simulink model "PubIfDecisionTOS_MDL"  (R2020b)
settings: configuration reference "DspaceConfig" (kept outside this file)
PostLoadFcn:
  | if any(exist('dsrtsu_mdlpostloadfcn', 'file') ~= 0), dsrtsu_mdlpostloadfcn('Execute', bdroot); end
InitFcn:
  | , if any(exist('dsmpb_private', 'file') ~= 0), dsmpb_private('dsmpb_mdlclblib', 'Init', bdroot); end,
undefined symbols (not defined in the file or in its folder): C_TOS_ACCEgoRAxletoFbumplength_m, C_TOS_ACCTargetFront_Flag, C_TOS_AEBJAPedObjDxThre_Val, C_TOS_AEBJAPedObjDyThre_Val, C_TOS_AEBJATargetSize_Val, C_TOS_AEBJAVehObjDxThre_Val, C_TOS_AEBJAVehObjDyThre_Val, C_TOS_AEBJuncPedTargetSize_Val, C_TOS_AEBLatObjDxThre_Val, C_TOS_AEBLatPedDyThre_Val, C_TOS_AEBLatTargetSize_Val, C_TOS_AEBLongTargetInEgoFront_Flag, C_TOS_axAbsGround_Parameter, C_TOS_CameraConfirmedFlag, C_TOS_CNsubjWidth, C_TOS_CurrentLaneCoreMinWidth_Val, C_TOS_CutInProb_Val_Zero, C_TOS_CutOutProb_Val_Zero, C_TOS_D2R_Val, C_TOS_DefaultValueObjectToCenterLine_dy, C_TOS_EgoCarWidth_Val, C_TOS_EgoDxRefPoint_m, C_TOS_EgoRAxletoFbumplength_m, C_TOS_HalfWidthVehicle_Con, C_TOS_HWA_CurrentLaneFlag, C_TOS_HWA_LeftLaneFlag, C_TOS_HWA_MovingDir_Vaild, C_TOS_HWA_MovState_Vaild, C_TOS_HWA_RightLaneFlag, C_TOS_LaneLineCourseErrorFront, C_TOS_LaneLineCourseErrorRear, C_TOS_MotorbikeDefaultWidth_m, C_TOS_NumberOfEffectiveTargets, C_TOS_Obj_Age_Val, C_TOS_Objdx_Constraint_Val, C_TOS_ObjectDefaultWidth_m, C_TOS_ObjInCurrentLane_Val, C_TOS_ObjInCurrentLaneValid, C_TOS_ObjInLeftLaneValid, C_TOS_ObjInRightLaneValid, C_TOS_ObjNotInCurrentLane_Val, C_TOS_ObjNotREElementType, C_TOS_ObjPredictDis_dy_ConstantVal_Zeros, C_TOS_ObjToCenterLine_ConstantVal_Zeros, C_TOS_OFMObjIDInvilad_Val, C_TOS_PIL_LatDisCons_Val_zero, C_TOS_PIL_ObjectCutInFlag_b, C_TOS_PIL_ObjectCutOutFlag_b, C_TOS_PIL_ObjLaneProb_al_Val, C_TOS_PP_ObjFusType_FC_Confirm_b, C_TOS_PP_ObjFusType_FC_FR_Confirm_b, C_TOS_PP_ObjFusType_FR_Confirm_b, C_TOS_RE_80BoolDefault_Val, C_TOS_RE_80Single181Default_Val, C_TOS_RE_80Single255Default_Val, C_TOS_RE_80Uint8Default_Val, C_TOS_RE_D2R, C_TOS_RE_D_180_Val, C_TOS_RE_InvalidObjectID_Val, C_TOS_RE_InvalidTargetChainDir_Val ... (+142)
libraries: simulink x1650, TOS_LIB x361, canfdmsglib x14
(part 23 of 69)

== system PubIfDecisionTOS_MDL/TOS_20201112/TOS_2012080320/PIL_1029/BoundaryCalculat/Lane_BoundaryCalculat/Lane_Boundary/Boundary/LeftLane_Boundary ==
  note: 用左侧车道虚拟出，左车道相邻车道
  Object_DX : Inport
  C_LaneLineCourseErrorFront : Inport  Port=2
  C_LaneLineCourseErrorRear : Inport  Port=3
  PP_CurrentLaneWidth : Inport  Port=4
  PP_LeftLaneWidth : Inport  Port=5
  SameLane_CoreArea_Boundary : Inport  Port=6
  LeftLane_BasicLaneWidth : Inport  Port=7
  Constant3 : Constant  Value=C_TOS_CurrentLaneCoreMinWidth_Val  OutDataTypeStr=single
      settings: AttributesFormatString=C_TOS_CurrentLaneCoreMinWidth_Val = 0
  Gain{,1..5} (6 alike) : Gain  Gain=0.5  ParamDataTypeStr=single  OutDataTypeStr=single
  Math Function : Math  Operator=square  SignedPower=on  OutDataTypeStr=single  SaturateOnIntegerOverflow=on
  MinMax : MinMax  Function=max  Inputs=2
  Product : Product  OutDataTypeStr=single
  Subtract : Sum  Inputs=+-  OutDataTypeStr=single
  Subtract1 : Sum  OutDataTypeStr=single
  Subtract2 : Sum  Inputs=+-  OutDataTypeStr=single
  Subtract3 : Sum  OutDataTypeStr=single
  Subtract4 : Sum  Inputs=+-  OutDataTypeStr=single
  Switch1 : Switch  OutDataTypeStr=single
  LeftLane_CoreArea_Boundary : Outport  OutDataTypeStr=single
  LeftLane_EdgeLeft_Boundary : Outport  Port=2
  LeftLane_EdgeRight_Boundary : Outport  Port=3
  wires:
  SameLane_CoreArea_Boundary/1 -> Subtract2/2
  Gain5/1 -> Subtract3/2
  Subtract4/1 -> LeftLane_EdgeLeft_Boundary/1
  Subtract3/1 -> Subtract4/1
  Gain4/1 -> Subtract3/1
  [LeftLane_CoreArea_Boundary] -> Subtract4/2
  PP_CurrentLaneWidth/1 -> Gain2/1
  Subtract1/1 -> Subtract2/1
  Gain3/1 -> Subtract1/2
  Gain2/1 -> Subtract1/1
  PP_LeftLaneWidth/1 -> Gain3/1, Gain4/1, Gain5/1
  Subtract2/1 -> LeftLane_EdgeRight_Boundary/1
  C_LaneLineCourseErrorRear/1 -> Switch1/3
  Switch1/1 -> Product/1
  Subtract/1 -> MinMax/1
  Gain1/1 -> Subtract/1
  LeftLane_BasicLaneWidth/1 -> Gain1/1
  Product/1 -> Subtract/2
  Math Function/1 -> Gain/1
  Gain/1 -> Product/2
  C_LaneLineCourseErrorFront/1 -> Switch1/1
  Object_DX/1 -> Math Function/1, Switch1/2
  Constant3/1 -> MinMax/2
  MinMax/1 -> LeftLane_CoreArea_Boundary/1, [LeftLane_CoreArea_Boundary]

== system PubIfDecisionTOS_MDL/TOS_20201112/TOS_2012080320/PIL_1029/BoundaryCalculat/Lane_BoundaryCalculat/Lane_Boundary/Boundary/RightLane_BasicLaneWidth ==
  ObjectType : Inport
  object_MovingState : Inport  Port=2
  PP_RightLaneWidth : Inport  Port=3
  Compare To Constant1 : simulink/Logic and Bit Operations/Compare To Constant  relop===  const=OFM_OBJ_TYPE_E.CAR  OutDataTypeStr=boolean
      settings: AttributesFormatString=OFM_OBJ_TYPE_E.CAR = 2
  Compare To Constant10 : simulink/Logic and Bit Operations/Compare To Constant  relop===  const=OFM_OBJ_MOVINGSTATE_E.UNKNOWN  OutDataTypeStr=boolean
      settings: AttributesFormatString=OFM_OBJ_MOVINGSTATE_E.UNKNOWN = 1
  Compare To Constant2 : simulink/Logic and Bit Operations/Compare To Constant  relop===  const=OFM_OBJ_TYPE_E.TRUCK  OutDataTypeStr=boolean
      settings: AttributesFormatString=OFM_OBJ_TYPE_E.TRUCK = 3
  Compare To Constant3 : simulink/Logic and Bit Operations/Compare To Constant  relop===  const=OFM_OBJ_TYPE_E.MOTORBIKE  OutDataTypeStr=boolean
      settings: AttributesFormatString=OFM_OBJ_TYPE_E.MOTORBIKE = 4
  Compare To Constant4 : simulink/Logic and Bit Operations/Compare To Constant  relop===  const=OFM_OBJ_TYPE_E.PEDESTRIAN  OutDataTypeStr=boolean
      settings: AttributesFormatString=OFM_OBJ_TYPE_E.PEDESTRIAN = 6
  Compare To Constant5 : simulink/Logic and Bit Operations/Compare To Constant  relop===  const=OFM_OBJ_TYPE_E.BICYCLE  OutDataTypeStr=boolean
      settings: AttributesFormatString=OFM_OBJ_TYPE_E.BICYCLE = 5
  Compare To Constant6 : simulink/Logic and Bit Operations/Compare To Constant  relop===  const=OFM_OBJ_TYPE_E.UNKNOWN_TYPE  OutDataTypeStr=boolean
      settings: AttributesFormatString=OFM_OBJ_TYPE_E.UNKNOWN_TYPE = 1
  Compare To Constant7 : simulink/Logic and Bit Operations/Compare To Constant  relop===  const=OFM_OBJ_TYPE_E.GENERAL_OBJECT  OutDataTypeStr=boolean
      settings: AttributesFormatString=OFM_OBJ_TYPE_E.GENERAL_OBJECT = 7
  Compare To Constant8 : simulink/Logic and Bit Operations/Compare To Constant  relop===  const=OFM_OBJ_TYPE_E.ANIMAL  OutDataTypeStr=boolean
      settings: AttributesFormatString=OFM_OBJ_TYPE_E.ANIMAL = 8
  Compare To Constant9 : simulink/Logic and Bit Operations/Compare To Constant  relop===  const=OFM_OBJ_MOVINGSTATE_E.STATIONARY  OutDataTypeStr=boolean
      settings: AttributesFormatString=OFM_OBJ_MOVINGSTATE_E.STATIONARY = 3
  Constant1 : Constant  Value=P_TOS_BasicLaneWidth_CAR_MinVal  OutDataTypeStr=single
      settings: AttributesFormatString=P_TOS_BasicLaneWidth_CAR_MinVal = 2.5
  Constant2 : Constant  Value=P_TOS_BasicLaneWidth_Pedestrian_MinVal  OutDataTypeStr=single
      settings: AttributesFormatString=P_TOS_BasicLaneWidth_Pedestrian_MinVal = 2
  Constant3 : Constant  Value=P_TOS_BasicLaneWidth_Bicycle_MinVal  OutDataTypeStr=single
      settings: AttributesFormatString=P_TOS_BasicLaneWidth_Bicycle_MinVal = 2.2
  Constant4 : Constant  Value=P_TOS_BasicLaneWidth_OthertType_MinVal  OutDataTypeStr=single
      settings: AttributesFormatString=P_TOS_BasicLaneWidth_OthertType_MinVal = 2.0
  Constant5 : Constant  Value=P_TOS_BasicLaneWidth_OthertType_MinVal  OutDataTypeStr=single
      settings: AttributesFormatString=P_TOS_BasicLaneWidth_OthertType_MinVal = 2.0
  Constant6 : Constant  Value=P_TOS_BasicLaneWidth_StillObj_MinVal  OutDataTypeStr=single
      settings: AttributesFormatString=P_TOS_BasicLaneWidth_StillObj_MinVal = 1.9
  Data Type Conversion : DataTypeConversion  OutDataTypeStr=Enum: OFM_OBJ_TYPE_E
  Data Type Conversion1 : DataTypeConversion  OutDataTypeStr=Enum: OFM_OBJ_MOVINGSTATE_E
  Logical Operator1 : Logic  Operator=OR  Inputs=3  AllPortsSameDT=off  OutDataTypeStr=boolean
  Logical Operator2 : Logic  Operator=OR  Inputs=3  AllPortsSameDT=off  OutDataTypeStr=boolean
  Logical Operator3 : Logic  Operator=OR  AllPortsSameDT=off  OutDataTypeStr=boolean
  MinMax : MinMax  Inputs=2  OutDataTypeStr=single
  Switch{1..5} (5 alike) : Switch  Criteria=u2 > Threshold
  RightLane_BasicLaneWidth : Outport
  wires:
  ObjectType/1 -> Data Type Conversion/1
  object_MovingState/1 -> Data Type Conversion1/1
  Compare To Constant4/1 -> Switch2/2
  Constant1/1 -> Switch1/1
  Constant3/1 -> Switch3/1
  Compare To Constant5/1 -> Switch3/2
  Constant5/1 -> Switch4/3
  Data Type Conversion/1 -> Compare To Constant1/1, Compare To Constant2/1, Compare To Constant6/1, Compare To Constant8/1, Compare To Constant7/1, Compare To Constant5/1, Compare To Constant4/1, Compare To Constant3/1
  Constant4/1 -> Switch4/1
  Constant2/1 -> Switch2/1
  Switch2/1 -> Switch1/3
  Switch4/1 -> Switch3/3
  Switch3/1 -> Switch2/3
  Compare To Constant3/1 -> Logical Operator1/3
  Switch1/1 -> Switch5/3
  Compare To Constant1/1 -> Logical Operator1/1
  Compare To Constant7/1 -> Logical Operator2/2
  Logical Operator2/1 -> Switch4/2
  Compare To Constant6/1 -> Logical Operator2/1
  Compare To Constant8/1 -> Logical Operator2/3
  Logical Operator1/1 -> Switch1/2
  Data Type Conversion1/1 -> Compare To Constant9/1, Compare To Constant10/1
  Compare To Constant2/1 -> Logical Operator1/2
  PP_RightLaneWidth/1 -> MinMax/1
  MinMax/1 -> RightLane_BasicLaneWidth/1
  Compare To Constant10/1 -> Logical Operator3/2
  Compare To Constant9/1 -> Logical Operator3/1
  Logical Operator3/1 -> Switch5/2
  Constant6/1 -> Switch5/1
  Switch5/1 -> MinMax/2

== system PubIfDecisionTOS_MDL/TOS_20201112/TOS_2012080320/PIL_1029/BoundaryCalculat/Lane_BoundaryCalculat/Lane_Boundary/Boundary/RightLane_Boundary ==
  note: 用右侧车道虚拟出，右车道相邻车道
  Object_DX : Inport
  C_LaneLineCourseErrorFront : Inport  Port=2
  C_LaneLineCourseErrorRear : Inport  Port=3
  PP_CurrentLaneWidth : Inport  Port=4
  PP_RightLaneWidth : Inport  Port=5
  SameLane_CoreArea_Boundary : Inport  Port=6
  RightLane_BasicLaneWidth : Inport  Port=7
  Constant3 : Constant  Value=C_TOS_CurrentLaneCoreMinWidth_Val  OutDataTypeStr=single
      settings: AttributesFormatString=C_TOS_CurrentLaneCoreMinWidth_Val = 0
  Gain{,1..5} (6 alike) : Gain  Gain=0.5  ParamDataTypeStr=single  OutDataTypeStr=single
  Math Function : Math  Operator=square  SignedPower=on  OutDataTypeStr=single  SaturateOnIntegerOverflow=on
  MinMax : MinMax  Function=max  Inputs=2
  Product : Product  OutDataTypeStr=single
  Subtract : Sum  Inputs=+-  OutDataTypeStr=single
  Subtract1 : Sum  OutDataTypeStr=single
  Subtract2 : Sum  Inputs=+-  OutDataTypeStr=single
  Subtract3 : Sum  OutDataTypeStr=single
  Subtract4 : Sum  Inputs=+-  OutDataTypeStr=single
  Switch1 : Switch  OutDataTypeStr=single
  RightLane_CoreArea_Boundary : Outport  OutDataTypeStr=single
  RightLane_EdgeLeft_Boundary : Outport  Port=2
  RightLane_EdgeRight_Boundary : Outport  Port=3
  wires:
  Subtract2/1 -> RightLane_EdgeLeft_Boundary/1
  Subtract4/1 -> RightLane_EdgeRight_Boundary/1
  Gain5/1 -> Subtract3/2
  PP_CurrentLaneWidth/1 -> Gain2/1
  Gain4/1 -> Subtract3/1
  PP_RightLaneWidth/1 -> Gain5/1, Gain4/1, Gain3/1
  Subtract3/1 -> Subtract4/1
  [RightLane_CoreArea_Boundary] -> Subtract4/2
  Subtract1/1 -> Subtract2/1
  Gain3/1 -> Subtract1/2
  Gain2/1 -> Subtract1/1
  SameLane_CoreArea_Boundary/1 -> Subtract2/2
  C_LaneLineCourseErrorRear/1 -> Switch1/3
  Switch1/1 -> Product/1
  Subtract/1 -> MinMax/1
  Gain1/1 -> Subtract/1
  RightLane_BasicLaneWidth/1 -> Gain1/1
  Product/1 -> Subtract/2
  Math Function/1 -> Gain/1
  Gain/1 -> Product/2
  C_LaneLineCourseErrorFront/1 -> Switch1/1
  Object_DX/1 -> Math Function/1, Switch1/2
  Constant3/1 -> MinMax/2
  MinMax/1 -> RightLane_CoreArea_Boundary/1, [RightLane_CoreArea_Boundary]

== system PubIfDecisionTOS_MDL/TOS_20201112/TOS_2012080320/PIL_1029/BoundaryCalculat/Lane_BoundaryCalculat/Lane_Boundary/Boundary/SameLane_BasicLaneWidth ==
  ObjectType : Inport
  object_MovingState : Inport  Port=2
  PP_CurrentLaneWidth : Inport  Port=3
  Compare To Constant1 : simulink/Logic and Bit Operations/Compare To Constant  relop===  const=OFM_OBJ_TYPE_E.CAR  OutDataTypeStr=boolean
      settings: AttributesFormatString=OFM_OBJ_TYPE_E.CAR = 2
  Compare To Constant10 : simulink/Logic and Bit Operations/Compare To Constant  relop===  const=OFM_OBJ_MOVINGSTATE_E.UNKNOWN  OutDataTypeStr=boolean
      settings: AttributesFormatString=OFM_OBJ_MOVINGSTATE_E.UNKNOWN = 1
  Compare To Constant2 : simulink/Logic and Bit Operations/Compare To Constant  relop===  const=OFM_OBJ_TYPE_E.TRUCK  OutDataTypeStr=boolean
      settings: AttributesFormatString=OFM_OBJ_TYPE_E.TRUCK = 3
  Compare To Constant3 : simulink/Logic and Bit Operations/Compare To Constant  relop===  const=OFM_OBJ_TYPE_E.MOTORBIKE  OutDataTypeStr=boolean
      settings: AttributesFormatString=OFM_OBJ_TYPE_E.MOTORBIKE = 4
  Compare To Constant4 : simulink/Logic and Bit Operations/Compare To Constant  relop===  const=OFM_OBJ_TYPE_E.PEDESTRIAN  OutDataTypeStr=boolean
      settings: AttributesFormatString=OFM_OBJ_TYPE_E.PEDESTRIAN = 6
  Compare To Constant5 : simulink/Logic and Bit Operations/Compare To Constant  relop===  const=OFM_OBJ_TYPE_E.BICYCLE  OutDataTypeStr=boolean
      settings: AttributesFormatString=OFM_OBJ_TYPE_E.BICYCLE = 5
  Compare To Constant6 : simulink/Logic and Bit Operations/Compare To Constant  relop===  const=OFM_OBJ_TYPE_E.UNKNOWN_TYPE  OutDataTypeStr=boolean
      settings: AttributesFormatString=OFM_OBJ_TYPE_E.UNKNOWN_TYPE = 1
  Compare To Constant7 : simulink/Logic and Bit Operations/Compare To Constant  relop===  const=OFM_OBJ_TYPE_E.GENERAL_OBJECT  OutDataTypeStr=boolean
      settings: AttributesFormatString=OFM_OBJ_TYPE_E.GENERAL_OBJECT = 7
  Compare To Constant8 : simulink/Logic and Bit Operations/Compare To Constant  relop===  const=OFM_OBJ_TYPE_E.ANIMAL  OutDataTypeStr=boolean
      settings: AttributesFormatString=OFM_OBJ_TYPE_E.ANIMAL = 8
  Compare To Constant9 : simulink/Logic and Bit Operations/Compare To Constant  relop===  const=OFM_OBJ_MOVINGSTATE_E.STATIONARY  OutDataTypeStr=boolean
      settings: AttributesFormatString=OFM_OBJ_MOVINGSTATE_E.STATIONARY = 3
  Constant1 : Constant  Value=P_TOS_BasicLaneWidth_CAR_MinVal  OutDataTypeStr=single
      settings: AttributesFormatString=P_TOS_BasicLaneWidth_CAR_MinVal = 2.5
  Constant2 : Constant  Value=P_TOS_BasicLaneWidth_Pedestrian_MinVal  OutDataTypeStr=single
      settings: AttributesFormatString=P_TOS_BasicLaneWidth_Pedestrian_MinVal = 2
  Constant3 : Constant  Value=P_TOS_BasicLaneWidth_Bicycle_MinVal  OutDataTypeStr=single
      settings: AttributesFormatString=P_TOS_BasicLaneWidth_Bicycle_MinVal = 2.2
  Constant4 : Constant  Value=P_TOS_BasicLaneWidth_OthertType_MinVal  OutDataTypeStr=single
      settings: AttributesFormatString=P_TOS_BasicLaneWidth_OthertType_MinVal = 2.0
  Constant5 : Constant  Value=P_TOS_BasicLaneWidth_OthertType_MinVal  OutDataTypeStr=single
      settings: AttributesFormatString=P_TOS_BasicLaneWidth_OthertType_MinVal = 2.0
  Constant6 : Constant  Value=P_TOS_BasicLaneWidth_StillObj_MinVal  OutDataTypeStr=single
      settings: AttributesFormatString=P_TOS_BasicLaneWidth_StillObj_MinVal = 1.9
  Data Type Conversion : DataTypeConversion  OutDataTypeStr=Enum: OFM_OBJ_TYPE_E
  Data Type Conversion1 : DataTypeConversion  OutDataTypeStr=Enum: OFM_OBJ_MOVINGSTATE_E
  Logical Operator1 : Logic  Operator=OR  Inputs=3  AllPortsSameDT=off  OutDataTypeStr=boolean
  Logical Operator2 : Logic  Operator=OR  Inputs=3  AllPortsSameDT=off  OutDataTypeStr=boolean
  Logical Operator3 : Logic  Operator=OR  AllPortsSameDT=off  OutDataTypeStr=boolean
  MinMax : MinMax  Inputs=2  OutDataTypeStr=single
  Switch{1..5} (5 alike) : Switch  Criteria=u2 > Threshold
  BasicLaneWidthOfCurrentLane : Outport
  wires:
  ObjectType/1 -> Data Type Conversion/1
  object_MovingState/1 -> Data Type Conversion1/1
  Compare To Constant4/1 -> Switch2/2
  Constant1/1 -> Switch1/1
  Constant3/1 -> Switch3/1
  Compare To Constant5/1 -> Switch3/2
  Constant5/1 -> Switch4/3
  Data Type Conversion/1 -> Compare To Constant1/1, Compare To Constant2/1, Compare To Constant6/1, Compare To Constant8/1, Compare To Constant7/1, Compare To Constant5/1, Compare To Constant4/1, Compare To Constant3/1
  Constant4/1 -> Switch4/1
  Constant2/1 -> Switch2/1
  Switch2/1 -> Switch1/3
  Switch4/1 -> Switch3/3
  Switch3/1 -> Switch2/3
  Compare To Constant3/1 -> Logical Operator1/3
  Switch1/1 -> Switch5/3
  Compare To Constant1/1 -> Logical Operator1/1
  Compare To Constant7/1 -> Logical Operator2/2
  Logical Operator2/1 -> Switch4/2
  Compare To Constant6/1 -> Logical Operator2/1
  Compare To Constant8/1 -> Logical Operator2/3
  Logical Operator1/1 -> Switch1/2
  Data Type Conversion1/1 -> Compare To Constant9/1, Compare To Constant10/1
  Compare To Constant2/1 -> Logical Operator1/2
  PP_CurrentLaneWidth/1 -> MinMax/1
  MinMax/1 -> BasicLaneWidthOfCurrentLane/1
  Compare To Constant10/1 -> Logical Operator3/2
  Compare To Constant9/1 -> Logical Operator3/1
  Logical Operator3/1 -> Switch5/2
  Constant6/1 -> Switch5/1
  Switch5/1 -> MinMax/2

== system PubIfDecisionTOS_MDL/TOS_20201112/TOS_2012080320/PIL_1029/BoundaryCalculat/Lane_BoundaryCalculat/Lane_Boundary/Boundary/SameLane_Boundary ==
  Object_DX : Inport
  C_LaneLineCourseErrorFront : Inport  Port=2
  C_LaneLineCourseErrorRear : Inport  Port=3
  PP_CurrentLaneWidth : Inport  Port=4
  PP_LeftLaneWidth : Inport  Port=5
  PP_RightLaneWidth : Inport  Port=6
  LeftLane_CoreArea_Boundary : Inport  Port=7
  RightLane_CoreArea_Boundary : Inport  Port=8
  SameLane_BasicLaneWidth : Inport  Port=9
  Constant3 : Constant  Value=C_TOS_CurrentLaneCoreMinWidth_Val  OutDataTypeStr=single
      settings: AttributesFormatString=C_TOS_CurrentLaneCoreMinWidth_Val = 0
  Gain{,1..5} (6 alike) : Gain  Gain=0.5  ParamDataTypeStr=single  OutDataTypeStr=single
  Math Function : Math  Operator=square  SignedPower=on  OutDataTypeStr=single  SaturateOnIntegerOverflow=on
  MinMax : MinMax  Function=max  Inputs=2
  Product : Product  OutDataTypeStr=single
  Subtract : Sum  Inputs=+-  OutDataTypeStr=single
  Subtract1 : Sum  OutDataTypeStr=single
  Subtract2 : Sum  Inputs=+-  OutDataTypeStr=single
  Subtract3 : Sum  OutDataTypeStr=single
  Subtract4 : Sum  Inputs=+-  OutDataTypeStr=single
  Switch1 : Switch  OutDataTypeStr=single
  SameLane_CoreArea_Boundary : Outport  OutDataTypeStr=single
  SameLane_EdgeLeft_Boundary : Outport  Port=2
  SameLane_EdgeRight_Boundary : Outport  Port=3
  wires:
  Subtract1/1 -> Subtract2/1
  PP_RightLaneWidth/1 -> Gain5/1
  Subtract2/1 -> SameLane_EdgeLeft_Boundary/1
  Gain3/1 -> Subtract1/2
  Gain5/1 -> Subtract3/2
  PP_CurrentLaneWidth/1 -> Gain4/1, Gain2/1
  LeftLane_CoreArea_Boundary/1 -> Subtract2/2
  Gain4/1 -> Subtract3/1
  Subtract4/1 -> SameLane_EdgeRight_Boundary/1
  Subtract3/1 -> Subtract4/1
  PP_LeftLaneWidth/1 -> Gain3/1
  RightLane_CoreArea_Boundary/1 -> Subtract4/2
  Gain2/1 -> Subtract1/1
  MinMax/1 -> SameLane_CoreArea_Boundary/1
  Constant3/1 -> MinMax/2
  Object_DX/1 -> Switch1/2, Math Function/1
  C_LaneLineCourseErrorFront/1 -> Switch1/1
  Gain/1 -> Product/2
  Math Function/1 -> Gain/1
  Product/1 -> Subtract/2
  SameLane_BasicLaneWidth/1 -> Gain1/1
  Gain1/1 -> Subtract/1
  Subtract/1 -> MinMax/1
  Switch1/1 -> Product/1
  C_LaneLineCourseErrorRear/1 -> Switch1/3

== system PubIfDecisionTOS_MDL/TOS_20201112/TOS_2012080320/PIL_1029/BoundaryCalculat/ObjectToCenterLine_dyc/LeftLane/LeftCenterLine_dyc/ObjToCenterLine_dyc_LeftLane ==
  Object_DY : Inport
  Object_DX : Inport  Port=2
  line01_C0 : Inport  Port=3
  line01_C1 : Inport  Port=4
  line01_C2 : Inport  Port=5
  line01_C3 : Inport  Port=6
  line01_dDisStart : Inport  Port=7
  line01_dDisEnd : Inport  Port=8
  line02_C0 : Inport  Port=9
  line02_C1 : Inport  Port=10
  line02_C2 : Inport  Port=11
  line02_C3 : Inport  Port=12
  line02_dDisStart : Inport  Port=13
  line02_dDisEnd : Inport  Port=14
  line03_C0 : Inport  Port=15
  line03_C1 : Inport  Port=16
  line03_C2 : Inport  Port=17
  line03_C3 : Inport  Port=18
  line03_dDisStart : Inport  Port=19
  line03_dDisEnd : Inport  Port=20
  line04_C0 : Inport  Port=21
  line04_C1 : Inport  Port=22
  line04_C2 : Inport  Port=23
  line04_C3 : Inport  Port=24
  line04_dDisStart : Inport  Port=25
  line04_dDisEnd : Inport  Port=26
  line05_C0 : Inport  Port=27
  line05_C1 : Inport  Port=28
  line05_C2 : Inport  Port=29
  line05_C3 : Inport  Port=30
  line05_dDisStart : Inport  Port=31
  line05_dDisEnd : Inport  Port=32
  line06_C0 : Inport  Port=33
  line06_C1 : Inport  Port=34
  line06_C2 : Inport  Port=35
  line06_C3 : Inport  Port=36
  line06_dDisStart : Inport  Port=37
  line06_dDisEnd : Inport  Port=38
  Action Port : ActionPort  ActionPortLabel=else
  Constant1 : Constant  Value=C_TOS_DefaultValueObjectToCenterLine_dy  OutDataTypeStr=single
      settings: AttributesFormatString=C_TOS_DefaultValueObjectToCenterLine_dy = 255
  Subtract : Sum  Inputs=+-
  Switch{,1..5} (6 alike) : Switch  Criteria=u2 ~= 0
  line01_DisJudge : Subsystem
  line01_dy : Subsystem
  line02_DisJudge : Subsystem
  line02_dy : Subsystem
  line03_DisJudge : Subsystem
  line03_dy : Subsystem
  line04_DisJudge : Subsystem
  line04_dy : Subsystem
  line05_DisJudge : Subsystem
  line05_dy : Subsystem
  line06_DisJudge : Subsystem
  line06_dy : Subsystem
  ObjectToCenterLine_dyc_LeftLane : Outport
  wires:
  Subtract/1 -> ObjectToCenterLine_dyc_LeftLane/1
  Object_DX/1 -> line01_dy/1(Object_DX), [Object_DX]
  line02_dDisEnd/1 -> line02_DisJudge/3(line02_dDisEnd)
  [Object_DX] -> line06_DisJudge/1(Object_DX)
  line05_dDisEnd/1 -> line05_DisJudge/3(line05_dDisEnd)
  line05_C0/1 -> line05_dy/2(line05_C0)
  line04_dDisEnd/1 -> line04_DisJudge/3(line04_dDisEnd)
  line06_dDisStart/1 -> line06_DisJudge/2(line06_dDisStart)
  line01_C0/1 -> line01_dy/2(line01_C0)
  [Object_DX] -> line05_DisJudge/1(Object_DX)
  [Object_DX] -> line04_DisJudge/1(Object_DX)
  line05_dy/1(line05_dy) -> Switch4/1
  [Object_DX] -> line01_DisJudge/1(Object_DX)
  line01_dDisEnd/1 -> line01_DisJudge/3(line01_dDisEnd)
  [Object_DX] -> line03_dy/1(Object_DX)
  line01_C1/1 -> line01_dy/3(line01_C1)
  line04_C0/1 -> line04_dy/2(line04_C0)
  line04_dDisStart/1 -> line04_DisJudge/2(line04_dDisStart)
  Constant1/1 -> Switch5/3
  line03_dDisStart/1 -> line03_DisJudge/2(line03_dDisStart)
  Switch/1 -> Subtract/2
  line02_dDisStart/1 -> line02_DisJudge/2(line02_dDisStart)
  line06_C3/1 -> line06_dy/5(line6_C3)
  line06_C0/1 -> line06_dy/2(line06_C0)
  line03_C1/1 -> line03_dy/3(line03_C1)
  line01_dDisStart/1 -> line01_DisJudge/2(line01_dDisStart)
  [Object_DX] -> line03_DisJudge/1(Object_DX)
  line06_C1/1 -> line06_dy/3(line06_C1)
  Switch5/1 -> Switch4/3
  line05_DisJudge/1(line05_DisJudge) -> Switch4/2
  line03_DisJudge/1(line03_DisJudge) -> Switch2/2
  line02_dy/1(line02_dy) -> Switch1/1
  line03_dy/1(line03_dy) -> Switch2/1
  line06_DisJudge/1(line06_DisJudge) -> Switch5/2
  Switch3/1 -> Switch2/3
  line04_dy/1(line04_dy) -> Switch3/1
  line02_C3/1 -> line02_dy/5(line02_C3)
  line04_DisJudge/1(line04_DisJudge) -> Switch3/2
  line04_C1/1 -> line04_dy/3(line04_C1)
  [Object_DX] -> line02_dy/1(Object_DX)
  line04_C3/1 -> line04_dy/5(line04_C3)
  line01_C2/1 -> line01_dy/4(line01_C2)
  line06_dDisEnd/1 -> line06_DisJudge/3(line06_dDisEnd)
  line01_DisJudge/1(line01_DisJudge) -> Switch/2
  Switch4/1 -> Switch3/3
  Object_DY/1 -> Subtract/1
  line01_dy/1(line01_dy) -> Switch/1
  [Object_DX] -> line02_DisJudge/1(Object_DX)
  line06_dy/1(line6_dy) -> Switch5/1
  line06_C2/1 -> line06_dy/4(line06_C2)
  line05_C1/1 -> line05_dy/3(line05_C1)
  line03_C2/1 -> line03_dy/4(line03_C2)
  line05_dDisStart/1 -> line05_DisJudge/2(line05_dDisStart)
  line02_C2/1 -> line02_dy/4(line02_C2)
  line02_C0/1 -> line02_dy/2(line02_C0)
  Switch2/1 -> Switch1/3
  line05_C3/1 -> line05_dy/5(line05_C3)
  [Object_DX] -> line06_dy/1(Object_DX)
  line03_dDisEnd/1 -> line03_DisJudge/3(line03_dDisEnd)
  line04_C2/1 -> line04_dy/4(line04_C2)
  Switch1/1 -> Switch/3
  [Object_DX] -> line04_dy/1(Object_DX)
  [Object_DX] -> line05_dy/1(Object_DX)
  line03_C3/1 -> line03_dy/5(line03_C3)
  line02_DisJudge/1(line02_DisJudge) -> Switch1/2
  line05_C2/1 -> line05_dy/4(line05_C2)
  line02_C1/1 -> line02_dy/3(line02_C1)
  line01_C3/1 -> line01_dy/5(line01_C3)
  line03_C0/1 -> line03_dy/2(line03_C0)

== system PubIfDecisionTOS_MDL/TOS_20201112/TOS_2012080320/PIL_1029/BoundaryCalculat/ObjectToCenterLine_dyc/LeftLane/LeftCenterLine_dyc/ObjToCenterLine_dyc_LeftLaneDefault ==
  Action Port : ActionPort  ActionPortLabel=if(u1 ~= 0)
  Constant2 : Constant  Value=255  OutDataTypeStr=single
  ObjectToCenterLine_dyc_LeftLane : Outport
  wires:
  Constant2/1 -> ObjectToCenterLine_dyc_LeftLane/1

== system PubIfDecisionTOS_MDL/TOS_20201112/TOS_2012080320/PIL_1029/BoundaryCalculat/ObjectToCenterLine_dyc/LeftLane/PIL_ObjectToCenterLine_dy_Filt/PIL_ObjectToCenterLine_dy ==
  ObjectID_Filt_K1 : Inport
  ObjectToCenterLine_dy_Filt_K1 : Inport  Port=2  OutDataTypeStr=single
  ObjectToCenterLine_dy : Inport  Port=3  OutDataTypeStr=single  Partition=on  PartitionDimension=1  PartitionWidth=1  PartitionOffset=0
  TOS_OFMObjValid_Flag : Inport  Port=4  OutDataTypeStr=uint8  Partition=on  PartitionDimension=1  PartitionWidth=1  PartitionOffset=0
  Object_ID : Inport  Port=5  OutDataTypeStr=uint8  Partition=on  PartitionDimension=1  PartitionWidth=1  PartitionOffset=0
  Object_Age : Inport  Port=6  Partition=on  PartitionDimension=1  PartitionWidth=1  PartitionOffset=0
  Compare To Constant : simulink/Logic and Bit Operations/Compare To Constant  relop===  const=C_TOS_OFMObjIDInvilad_Val  OutDataTypeStr=boolean
      settings: AttributesFormatString=C_TOS_OFMObjIDInvilad_Val = 0
  For Each : ForEach  DisableCoverage=on
  If : If  IfExpression=u1 ~= 0
  Merge : Merge
  Merge1 : Merge
  PP_SignalProcessingDefault : Subsystem  TreatAsAtomicUnit=on
  Subsystem : Subsystem
  Obj_ID : Outport  ConcatenationDimension=1
  ObjectToCenterLine_dy_Filt : Outport  Port=2  OutDataTypeStr=single  ConcatenationDimension=1
  wires:
  [TOS_OFMObjValid_Flag] -> Subsystem/6(TOS_OFMObjValid_Flag)
  TOS_OFMObjValid_Flag/1 -> Compare To Constant/1, [TOS_OFMObjValid_Flag]
  Object_Age/1 -> Subsystem/5(Object_Age)
  Merge/1 -> Obj_ID/1
  Merge1/1 -> ObjectToCenterLine_dy_Filt/1
  PP_SignalProcessingDefault/2(ObjectToCenterLine_dy_Filt) -> Merge1/1
  PP_SignalProcessingDefault/1(Obj_ID) -> Merge/1
  Subsystem/2(ObjectToCenterLine_dy_Filt) -> Merge1/2
  Subsystem/1(Obj_ID) -> Merge/2
  ObjectToCenterLine_dy/1 -> Subsystem/3(ObjectToCenterLine_dy)
  ObjectToCenterLine_dy_Filt_K1/1 -> Subsystem/2(ObjectToCenterLine_dy_Filt_K1)
  ObjectID_Filt_K1/1 -> Subsystem/1(ObjectID_Filt_K1)
  Compare To Constant/1 -> If/1
  Object_ID/1 -> Subsystem/4(Object_ID)
  If/1 -> PP_SignalProcessingDefault/Action
  If/2 -> Subsystem/Action

== system PubIfDecisionTOS_MDL/TOS_20201112/TOS_2012080320/PIL_1029/BoundaryCalculat/ObjectToCenterLine_dyc/RightLane/PIL_ObjectToCenterLine_dy_Filt/PIL_ObjectToCenterLine_dy ==
  ObjectID_Filt_K1 : Inport
  ObjectToCenterLine_dy_Filt_K1 : Inport  Port=2  OutDataTypeStr=single
  ObjectToCenterLine_dy : Inport  Port=3  OutDataTypeStr=single  Partition=on  PartitionDimension=1  PartitionWidth=1  PartitionOffset=0
  TOS_OFMObjValid_Flag : Inport  Port=4  OutDataTypeStr=uint8  Partition=on  PartitionDimension=1  PartitionWidth=1  PartitionOffset=0
  Object_ID : Inport  Port=5  OutDataTypeStr=uint8  Partition=on  PartitionDimension=1  PartitionWidth=1  PartitionOffset=0
  Object_Age : Inport  Port=6  Partition=on  PartitionDimension=1  PartitionWidth=1  PartitionOffset=0
  Compare To Constant : simulink/Logic and Bit Operations/Compare To Constant  relop===  const=C_TOS_OFMObjIDInvilad_Val  OutDataTypeStr=boolean
      settings: AttributesFormatString=C_TOS_OFMObjIDInvilad_Val = 0
  For Each : ForEach  DisableCoverage=on
  If : If  IfExpression=u1 ~= 0
  Merge : Merge
  Merge1 : Merge
  PP_SignalProcessingDefault : Subsystem  TreatAsAtomicUnit=on
  Subsystem : Subsystem
  Obj_ID : Outport  ConcatenationDimension=1
  ObjectToCenterLine_dy_Filt : Outport  Port=2  OutDataTypeStr=single  ConcatenationDimension=1
  wires:
  [TOS_OFMObjValid_Flag] -> Subsystem/6(TOS_OFMObjValid_Flag)
  TOS_OFMObjValid_Flag/1 -> Compare To Constant/1, [TOS_OFMObjValid_Flag]
  Object_Age/1 -> Subsystem/5(Object_Age)
  Merge/1 -> Obj_ID/1
  Merge1/1 -> ObjectToCenterLine_dy_Filt/1
  PP_SignalProcessingDefault/2(ObjectToCenterLine_dy_Filt) -> Merge1/1
  PP_SignalProcessingDefault/1(Obj_ID) -> Merge/1
  Subsystem/2(ObjectToCenterLine_dy_Filt) -> Merge1/2
  Subsystem/1(Obj_ID) -> Merge/2
  ObjectToCenterLine_dy/1 -> Subsystem/3(ObjectToCenterLine_dy)
  ObjectToCenterLine_dy_Filt_K1/1 -> Subsystem/2(ObjectToCenterLine_dy_Filt_K1)
  ObjectID_Filt_K1/1 -> Subsystem/1(ObjectID_Filt_K1)
  Compare To Constant/1 -> If/1
  Object_ID/1 -> Subsystem/4(Object_ID)
  If/1 -> PP_SignalProcessingDefault/Action
  If/2 -> Subsystem/Action

== system PubIfDecisionTOS_MDL/TOS_20201112/TOS_2012080320/PIL_1029/BoundaryCalculat/ObjectToCenterLine_dyc/RightLane/RightCenterLine_dyc/ObjToCenterLine_dyc_RightLane ==
  Object_DY : Inport
  Object_DX : Inport  Port=2
  line01_C0 : Inport  Port=3
  line01_C1 : Inport  Port=4
  line01_C2 : Inport  Port=5
  line01_C3 : Inport  Port=6
  line01_dDisStart : Inport  Port=7
  line01_dDisEnd : Inport  Port=8
  line02_C0 : Inport  Port=9
  line02_C1 : Inport  Port=10
  line02_C2 : Inport  Port=11
  line02_C3 : Inport  Port=12
  line02_dDisStart : Inport  Port=13
  line02_dDisEnd : Inport  Port=14
  line03_C0 : Inport  Port=15
  line03_C1 : Inport  Port=16
  line03_C2 : Inport  Port=17
  line03_C3 : Inport  Port=18
  line03_dDisStart : Inport  Port=19
  line03_dDisEnd : Inport  Port=20
  line04_C0 : Inport  Port=21
  line04_C1 : Inport  Port=22
  line04_C2 : Inport  Port=23
  line04_C3 : Inport  Port=24
  line04_dDisStart : Inport  Port=25
  line04_dDisEnd : Inport  Port=26
  line05_C0 : Inport  Port=27
  line05_C1 : Inport  Port=28
  line05_C2 : Inport  Port=29
  line05_C3 : Inport  Port=30
  line05_dDisStart : Inport  Port=31
  line05_dDisEnd : Inport  Port=32
  line06_C0 : Inport  Port=33
  line06_C1 : Inport  Port=34
  line06_C2 : Inport  Port=35
  line06_C3 : Inport  Port=36
  line06_dDisStart : Inport  Port=37
  line06_dDisEnd : Inport  Port=38
  Action Port : ActionPort  ActionPortLabel=else
  Constant1 : Constant  Value=C_TOS_DefaultValueObjectToCenterLine_dy  OutDataTypeStr=single
      settings: AttributesFormatString=C_TOS_DefaultValueObjectToCenterLine_dy = 255
  Subtract : Sum  Inputs=+-
  Switch{,1..5} (6 alike) : Switch  Criteria=u2 ~= 0
  line01_DisJudge : Subsystem
  line01_dy : Subsystem
  line02_DisJudge : Subsystem
  line02_dy : Subsystem
  line03_DisJudge : Subsystem
  line03_dy : Subsystem
  line04_DisJudge : Subsystem
  line04_dy : Subsystem
  line05_DisJudge : Subsystem
  line05_dy : Subsystem
  line06_DisJudge : Subsystem
  line06_dy : Subsystem
  ObjectToCenterLine_dyc_RightLane : Outport
  wires:
  line03_C0/1 -> line03_dy/2(line03_C0)
  line01_C3/1 -> line01_dy/5(line01_C3)
  line02_C1/1 -> line02_dy/3(line02_C1)
  line05_C2/1 -> line05_dy/4(line05_C2)
  line02_DisJudge/1(line02_DisJudge) -> Switch1/2
  line03_C3/1 -> line03_dy/5(line03_C3)
  [Object_DX] -> line05_dy/1(Object_DX)
  [Object_DX] -> line04_dy/1(Object_DX)
  Switch1/1 -> Switch/3
  line04_C2/1 -> line04_dy/4(line04_C2)
  line03_dDisEnd/1 -> line03_DisJudge/3(line03_dDisEnd)
  [Object_DX] -> line06_dy/1(Object_DX)
  line05_C3/1 -> line05_dy/5(line05_C3)
  Switch2/1 -> Switch1/3
  line02_C0/1 -> line02_dy/2(line02_C0)
  line02_C2/1 -> line02_dy/4(line02_C2)
  line05_dDisStart/1 -> line05_DisJudge/2(line05_dDisStart)
  line03_C2/1 -> line03_dy/4(line03_C2)
  line05_C1/1 -> line05_dy/3(line05_C1)
  line06_C2/1 -> line06_dy/4(line06_C2)
  line06_dy/1(line6_dy) -> Switch5/1
  [Object_DX] -> line02_DisJudge/1(Object_DX)
  line01_dy/1(line01_dy) -> Switch/1
  Object_DY/1 -> Subtract/1
  Switch4/1 -> Switch3/3
  line01_DisJudge/1(line01_DisJudge) -> Switch/2
  line06_dDisEnd/1 -> line06_DisJudge/3(line06_dDisEnd)
  line01_C2/1 -> line01_dy/4(line01_C2)
  line04_C3/1 -> line04_dy/5(line04_C3)
  [Object_DX] -> line02_dy/1(Object_DX)
  line04_C1/1 -> line04_dy/3(line04_C1)
  line04_DisJudge/1(line04_DisJudge) -> Switch3/2
  line02_C3/1 -> line02_dy/5(line02_C3)
  line04_dy/1(line04_dy) -> Switch3/1
  Switch3/1 -> Switch2/3
  line06_DisJudge/1(line06_DisJudge) -> Switch5/2
  line03_dy/1(line03_dy) -> Switch2/1
  line02_dy/1(line02_dy) -> Switch1/1
  line03_DisJudge/1(line03_DisJudge) -> Switch2/2
  line05_DisJudge/1(line05_DisJudge) -> Switch4/2
  Switch5/1 -> Switch4/3
  line06_C1/1 -> line06_dy/3(line06_C1)
  [Object_DX] -> line03_DisJudge/1(Object_DX)
  line01_dDisStart/1 -> line01_DisJudge/2(line01_dDisStart)
  line03_C1/1 -> line03_dy/3(line03_C1)
  line06_C0/1 -> line06_dy/2(line06_C0)
  line06_C3/1 -> line06_dy/5(line6_C3)
  line02_dDisStart/1 -> line02_DisJudge/2(line02_dDisStart)
  Switch/1 -> Subtract/2
  line03_dDisStart/1 -> line03_DisJudge/2(line03_dDisStart)
  Constant1/1 -> Switch5/3
  line04_dDisStart/1 -> line04_DisJudge/2(line04_dDisStart)
  line04_C0/1 -> line04_dy/2(line04_C0)
  line01_C1/1 -> line01_dy/3(line01_C1)
  [Object_DX] -> line03_dy/1(Object_DX)
  line01_dDisEnd/1 -> line01_DisJudge/3(line01_dDisEnd)
  [Object_DX] -> line01_DisJudge/1(Object_DX)
  line05_dy/1(line05_dy) -> Switch4/1
  [Object_DX] -> line04_DisJudge/1(Object_DX)
  [Object_DX] -> line05_DisJudge/1(Object_DX)
  line01_C0/1 -> line01_dy/2(line01_C0)
  line06_dDisStart/1 -> line06_DisJudge/2(line06_dDisStart)
  line04_dDisEnd/1 -> line04_DisJudge/3(line04_dDisEnd)
  line05_C0/1 -> line05_dy/2(line05_C0)
  line05_dDisEnd/1 -> line05_DisJudge/3(line05_dDisEnd)
  [Object_DX] -> line06_DisJudge/1(Object_DX)
  line02_dDisEnd/1 -> line02_DisJudge/3(line02_dDisEnd)
  Object_DX/1 -> [Object_DX], line01_dy/1(Object_DX)
  Subtract/1 -> ObjectToCenterLine_dyc_RightLane/1

== system PubIfDecisionTOS_MDL/TOS_20201112/TOS_2012080320/PIL_1029/BoundaryCalculat/ObjectToCenterLine_dyc/RightLane/RightCenterLine_dyc/ObjToCenterLine_dyc_RightLaneDefault ==
  Action Port : ActionPort  ActionPortLabel=if(u1 ~= 0)
  Constant2 : Constant  Value=255  OutDataTypeStr=single
  ObjectToCenterLine_dyc_LeftLane : Outport
  wires:
  Constant2/1 -> ObjectToCenterLine_dyc_LeftLane/1

== system PubIfDecisionTOS_MDL/TOS_20201112/TOS_2012080320/PIL_1029/BoundaryCalculat/ObjectToCenterLine_dyc/SameLane/PIL_ObjectToCenterLine_dy_Filt/PIL_ObjectToCenterLine_dy ==
  ObjectID_Filt_K1 : Inport
  ObjectToCenterLine_dy_Filt_K1 : Inport  Port=2  OutDataTypeStr=single
  ObjectToCenterLine_dy : Inport  Port=3  OutDataTypeStr=single  Partition=on  PartitionDimension=1  PartitionWidth=1  PartitionOffset=0
  TOS_OFMObjValid_Flag : Inport  Port=4  OutDataTypeStr=uint8  Partition=on  PartitionDimension=1  PartitionWidth=1  PartitionOffset=0
  Object_ID : Inport  Port=5  OutDataTypeStr=uint8  Partition=on  PartitionDimension=1  PartitionWidth=1  PartitionOffset=0
  Object_Age : Inport  Port=6  Partition=on  PartitionDimension=1  PartitionWidth=1  PartitionOffset=0
  Compare To Constant : simulink/Logic and Bit Operations/Compare To Constant  relop===  const=C_TOS_OFMObjIDInvilad_Val  OutDataTypeStr=boolean
      settings: AttributesFormatString=C_TOS_OFMObjIDInvilad_Val = 0
  For Each : ForEach  DisableCoverage=on
  If : If  IfExpression=u1 ~= 0
  Merge : Merge
  Merge1 : Merge
  PP_SignalProcessingDefault : Subsystem  TreatAsAtomicUnit=on
  Subsystem : Subsystem
  Obj_ID : Outport  ConcatenationDimension=1
  ObjectToCenterLine_dy_Filt : Outport  Port=2  OutDataTypeStr=single  ConcatenationDimension=1
  wires:
  [TOS_OFMObjValid_Flag] -> Subsystem/6(TOS_OFMObjValid_Flag)
  TOS_OFMObjValid_Flag/1 -> Compare To Constant/1, [TOS_OFMObjValid_Flag]
  Object_Age/1 -> Subsystem/5(Object_Age)
  Merge/1 -> Obj_ID/1
  Merge1/1 -> ObjectToCenterLine_dy_Filt/1
  PP_SignalProcessingDefault/2(ObjectToCenterLine_dy_Filt) -> Merge1/1
  PP_SignalProcessingDefault/1(Obj_ID) -> Merge/1
  Subsystem/2(ObjectToCenterLine_dy_Filt) -> Merge1/2
  Subsystem/1(Obj_ID) -> Merge/2
  ObjectToCenterLine_dy/1 -> Subsystem/3(ObjectToCenterLine_dy)
  ObjectToCenterLine_dy_Filt_K1/1 -> Subsystem/2(ObjectToCenterLine_dy_Filt_K1)
  ObjectID_Filt_K1/1 -> Subsystem/1(ObjectID_Filt_K1)
  Compare To Constant/1 -> If/1
  Object_ID/1 -> Subsystem/4(Object_ID)
  If/1 -> PP_SignalProcessingDefault/Action
  If/2 -> Subsystem/Action

== system PubIfDecisionTOS_MDL/TOS_20201112/TOS_2012080320/PIL_1029/BoundaryCalculat/ObjectToCenterLine_dyc/SameLane/SameCenterLine_dyc/ObjToCenterLine_dyc_CurrentLane ==
  Object_DY : Inport
  Object_DX : Inport  Port=2
  line01_C0 : Inport  Port=3
  line01_C1 : Inport  Port=4
  line01_C2 : Inport  Port=5
  line01_C3 : Inport  Port=6
  line01_dDisStart : Inport  Port=7
  line01_dDisEnd : Inport  Port=8
  line02_C0 : Inport  Port=9
  line02_C1 : Inport  Port=10
  line02_C2 : Inport  Port=11
  line02_C3 : Inport  Port=12
  line02_dDisStart : Inport  Port=13
  line02_dDisEnd : Inport  Port=14
  line03_C0 : Inport  Port=15
  line03_C1 : Inport  Port=16
  line03_C2 : Inport  Port=17
  line03_C3 : Inport  Port=18
  line03_dDisStart : Inport  Port=19
  line03_dDisEnd : Inport  Port=20
  line04_C0 : Inport  Port=21
  line04_C1 : Inport  Port=22
  line04_C2 : Inport  Port=23
  line04_C3 : Inport  Port=24
  line04_dDisStart : Inport  Port=25
  line04_dDisEnd : Inport  Port=26
  line05_C0 : Inport  Port=27
  line05_C1 : Inport  Port=28
  line05_C2 : Inport  Port=29
  line05_C3 : Inport  Port=30
  line05_dDisStart : Inport  Port=31
  line05_dDisEnd : Inport  Port=32
  line06_C0 : Inport  Port=33
  line06_C1 : Inport  Port=34
  line06_C2 : Inport  Port=35
  line06_C3 : Inport  Port=36
  line06_dDisStart : Inport  Port=37
  line06_dDisEnd : Inport  Port=38
  Action Port : ActionPort  ActionPortLabel=else
  Constant1 : Constant  Value=C_TOS_DefaultValueObjectToCenterLine_dy  OutDataTypeStr=single
      settings: AttributesFormatString=C_TOS_DefaultValueObjectToCenterLine_dy = 255
  Subtract : Sum  Inputs=+-
  Switch{,1..5} (6 alike) : Switch  Criteria=u2 ~= 0
  line01_DisJudge : Subsystem
  line01_dy : Subsystem
  line02_DisJudge : Subsystem
  line02_dy : Subsystem
  line03_DisJudge : Subsystem
  line03_dy : Subsystem
  line04_DisJudge : Subsystem
  line04_dy : Subsystem
  line05_DisJudge : Subsystem
  line05_dy : Subsystem
  line06_DisJudge : Subsystem
  line06_dy : Subsystem
  ObjectToCenterLine_dyc_CurrentLane : Outport
  wires:
  Subtract/1 -> ObjectToCenterLine_dyc_CurrentLane/1
  Object_DX/1 -> line01_dy/1(Object_DX), [Object_DX]
  line02_dDisEnd/1 -> line02_DisJudge/3(line02_dDisEnd)
  [Object_DX] -> line06_DisJudge/1(Object_DX)
  line05_dDisEnd/1 -> line05_DisJudge/3(line05_dDisEnd)
  line05_C0/1 -> line05_dy/2(line05_C0)
  line04_dDisEnd/1 -> line04_DisJudge/3(line04_dDisEnd)
  line06_dDisStart/1 -> line06_DisJudge/2(line06_dDisStart)
  line01_C0/1 -> line01_dy/2(line01_C0)
  [Object_DX] -> line05_DisJudge/1(Object_DX)
  [Object_DX] -> line04_DisJudge/1(Object_DX)
  line05_dy/1(line05_dy) -> Switch4/1
  [Object_DX] -> line01_DisJudge/1(Object_DX)
  line01_dDisEnd/1 -> line01_DisJudge/3(line01_dDisEnd)
  [Object_DX] -> line03_dy/1(Object_DX)
  line01_C1/1 -> line01_dy/3(line01_C1)
  line04_C0/1 -> line04_dy/2(line04_C0)
  line04_dDisStart/1 -> line04_DisJudge/2(line04_dDisStart)
  Constant1/1 -> Switch5/3
  line03_dDisStart/1 -> line03_DisJudge/2(line03_dDisStart)
  Switch/1 -> Subtract/2
  line02_dDisStart/1 -> line02_DisJudge/2(line02_dDisStart)
  line06_C3/1 -> line06_dy/5(line6_C3)
  line06_C0/1 -> line06_dy/2(line06_C0)
  line03_C1/1 -> line03_dy/3(line03_C1)
  line01_dDisStart/1 -> line01_DisJudge/2(line01_dDisStart)
  [Object_DX] -> line03_DisJudge/1(Object_DX)
  line06_C1/1 -> line06_dy/3(line06_C1)
  Switch5/1 -> Switch4/3
  line05_DisJudge/1(line05_DisJudge) -> Switch4/2
  line03_DisJudge/1(line03_DisJudge) -> Switch2/2
  line02_dy/1(line02_dy) -> Switch1/1
  line03_dy/1(line03_dy) -> Switch2/1
  line06_DisJudge/1(line06_DisJudge) -> Switch5/2
  Switch3/1 -> Switch2/3
  line04_dy/1(line04_dy) -> Switch3/1
  line02_C3/1 -> line02_dy/5(line02_C3)
  line04_DisJudge/1(line04_DisJudge) -> Switch3/2
  line04_C1/1 -> line04_dy/3(line04_C1)
  [Object_DX] -> line02_dy/1(Object_DX)
  line04_C3/1 -> line04_dy/5(line04_C3)
  line01_C2/1 -> line01_dy/4(line01_C2)
  line06_dDisEnd/1 -> line06_DisJudge/3(line06_dDisEnd)
  line01_DisJudge/1(line01_DisJudge) -> Switch/2
  Switch4/1 -> Switch3/3
  Object_DY/1 -> Subtract/1
  line01_dy/1(line01_dy) -> Switch/1
  [Object_DX] -> line02_DisJudge/1(Object_DX)
  line06_dy/1(line6_dy) -> Switch5/1
  line06_C2/1 -> line06_dy/4(line06_C2)
  line05_C1/1 -> line05_dy/3(line05_C1)
  line03_C2/1 -> line03_dy/4(line03_C2)
  line05_dDisStart/1 -> line05_DisJudge/2(line05_dDisStart)
  line02_C2/1 -> line02_dy/4(line02_C2)
  line02_C0/1 -> line02_dy/2(line02_C0)
  Switch2/1 -> Switch1/3
  line05_C3/1 -> line05_dy/5(line05_C3)
  [Object_DX] -> line06_dy/1(Object_DX)
  line03_dDisEnd/1 -> line03_DisJudge/3(line03_dDisEnd)
  line04_C2/1 -> line04_dy/4(line04_C2)
  Switch1/1 -> Switch/3
  [Object_DX] -> line04_dy/1(Object_DX)
  [Object_DX] -> line05_dy/1(Object_DX)
  line03_C3/1 -> line03_dy/5(line03_C3)
  line02_DisJudge/1(line02_DisJudge) -> Switch1/2
  line05_C2/1 -> line05_dy/4(line05_C2)
  line02_C1/1 -> line02_dy/3(line02_C1)
  line01_C3/1 -> line01_dy/5(line01_C3)
  line03_C0/1 -> line03_dy/2(line03_C0)

== system PubIfDecisionTOS_MDL/TOS_20201112/TOS_2012080320/PIL_1029/BoundaryCalculat/ObjectToCenterLine_dyc/SameLane/SameCenterLine_dyc/ObjToCenterLine_dyc_CurrentLaneDefault ==
  Action Port : ActionPort  ActionPortLabel=if(u1 ~= 0)
  Constant2 : Constant  Value=255  OutDataTypeStr=single
  ObjectToCenterLine_dyc_CurrentLane : Outport
  wires:
  Constant2/1 -> ObjectToCenterLine_dyc_CurrentLane/1

== system PubIfDecisionTOS_MDL/TOS_20201112/TOS_2012080320/PIL_1029/ObjCutInOut_Prob/ObjectCutIn/CutInProb_Calculate/CutInProb_Calculate_/CutInPredictDis_dy ==
  note: dx 修正vyc的 cut in 预测时间
  ObjectToCenterLine_dy_Filt : Inport  OutDataTypeStr=single
  ObjectToCenterLine_dy : Inport  Port=2  OutDataTypeStr=single
  ObjectType : Inport  Port=3
  Object_DX : Inport  Port=4
  PP_ObjectToCenterLine_vyc : Inport  Port=5
  CutInPredictTime : Subsystem
  CutInPredictTime_Constraint : Subsystem
  CutInPredictTime_Constraint2 : Subsystem
  PIL_CutInPredictTime_ObserVale : Outport  OutDataTypeStr=single
  PIL_CutInPredictTime_Constraint_ObserVale : Outport  Port=2  OutDataTypeStr=single
  CutInPredictDis_dy : Outport  Port=3  OutDataTypeStr=single
  wires:
  Object_DX/1 -> CutInPredictTime/5(Object_DX), CutInPredictTime_Constraint/2(Object_DX)
  ObjectToCenterLine_dy_Filt/1 -> CutInPredictTime/1(ObjectToCenterLine_dy_Filt)
  ObjectToCenterLine_dy/1 -> [ObjectToCenterLine_dy], CutInPredictTime/2(ObjectToCenterLine_dy)
  CutInPredictTime/1(CutInPredictTime) -> [PIL_CutInPredictTime_ObserVale], CutInPredictTime_Constraint/1(CutInPredictTime)
  CutInPredictTime_Constraint/1(CutInPredictTime_Constraint) -> [PIL_CutInPredictTime_Constraint_ObserVale], CutInPredictTime_Constraint2/2(CutInPredictTime_Constraint)
  PP_ObjectToCenterLine_vyc/1 -> CutInPredictTime_Constraint2/3(PP_ObjectToCenterLine_vyc), [PP_ObjectToCenterLine_vyc]
  CutInPredictTime_Constraint2/1(CutInPredictDis_dy) -> CutInPredictDis_dy/1
  [ObjectToCenterLine_dy] -> CutInPredictTime_Constraint2/1(ObjectToCenterLine_dy)
  ObjectType/1 -> CutInPredictTime/3(ObjectType)
  [PP_ObjectToCenterLine_vyc] -> CutInPredictTime/4(PP_ObjectToCenterLine_vyc)
  [PIL_CutInPredictTime_Constraint_ObserVale] -> PIL_CutInPredictTime_Constraint_ObserVale/1
  [PIL_CutInPredictTime_ObserVale] -> PIL_CutInPredictTime_ObserVale/1

== system PubIfDecisionTOS_MDL/TOS_20201112/TOS_2012080320/PIL_1029/ObjCutInOut_Prob/ObjectCutIn/CutInProb_Calculate/CutInProb_Calculate_/CutInProb ==
  CutInPredictDis_dy : Inport  OutDataTypeStr=single
  ObjectToCenterLine_dy : Inport  Port=2  OutDataTypeStr=single
  Object_Width : Inport  Port=3
  ObjectType : Inport  Port=4
  CutInObjWidthConstraint : Subsystem
  CutInProb_Calculation : Subsystem
  PIL_CutInPredictDis_dy_ObjWidthConstraint_ObserVale : Outport
  CutInProb : Outport  Port=2
  wires:
  ObjectType/1 -> CutInObjWidthConstraint/4(ObjectType)
  CutInPredictDis_dy/1 -> CutInObjWidthConstraint/1(CutInPredictDis_dy)
  ObjectToCenterLine_dy/1 -> CutInObjWidthConstraint/2(ObjectToCenterLine_dy)
  Object_Width/1 -> CutInObjWidthConstraint/3(Object_Width)
  CutInObjWidthConstraint/1(CutInPredictDis_dy_ObjWidthConstraint) -> [PIL_CutInPredictDis_dy_ObjWidthConstraint_ObserVale], CutInProb_Calculation/1(CutInPredictDis_dy_ObjWidthConstraint)
  CutInProb_Calculation/1(CutInProb_Calculation) -> CutInProb/1  "CutInProb"
  [PIL_CutInPredictDis_dy_ObjWidthConstraint_ObserVale] -> PIL_CutInPredictDis_dy_ObjWidthConstraint_ObserVale/1

== system PubIfDecisionTOS_MDL/TOS_20201112/TOS_2012080320/PIL_1029/ObjCutInOut_Prob/ObjectCutIn/CutInProb_Calculate/CutInProb_Calculate_/CutInProb_ScopeConstraint ==
  CutInProb : Inport  OutDataTypeStr=single
  PP_ObjectToCenterLine_vyc : Inport  Port=2  OutDataTypeStr=single
  ObjectToCenterLine_dy : Inport  Port=3  OutDataTypeStr=single
  PP_ObjectToCenterLine_dy : Inport  Port=4
  Object_Age : Inport  Port=5
  Object_Width : Inport  Port=6
  Abs : Abs
  Abs1 : Abs
  C_CutInProb_Val_Zero : Constant  Value=C_TOS_CutInProb_Val_Zero  OutDataTypeStr=single
      settings: AttributesFormatString=C_TOS_CutInProb_Val_Zero = 0
  Compare To Constant1 : simulink/Logic and Bit Operations/Compare To Constant  relop=>  const=P_TOS_ObjCutInObject_DY_Val  OutDataTypeStr=boolean
      settings: AttributesFormatString=P_TOS_ObjCutInObject_DY_Val = 2.4
  Compare To Constant2 : simulink/Logic and Bit Operations/Compare To Constant  relop=<  const=C_TOS_Obj_Age_Val  OutDataTypeStr=boolean
      settings: AttributesFormatString=C_TOS_Obj_Age_Val = 1
  Compare To Constant3 : simulink/Logic and Bit Operations/Compare To Constant  relop=<=  const=P_TOS_CutinObjvyThre_Val  OutDataTypeStr=boolean
      settings: AttributesFormatString=P_TOS_CutinObjvyThre_Val = 0.06
  CutInObjCutoutMov : Subsystem
  CutInObjWidthConstraint : Subsystem
  Logical Operator2 : Logic  Operator=OR  Inputs=4  AllPortsSameDT=off  OutDataTypeStr=boolean
  PP_ObjectToCenterLine_vyc1 : InportShadow  Port=2  OutDataTypeStr=single
  Switch1 : Switch  Criteria=u2 > Threshold  OutDataTypeStr=single
  Terminator : Terminator
  PIL_ObjectCutinMindFlg_ObserVale : Outport  OutDataTypeStr=boolean
  CutInProb_ScopeConstraint : Outport  Port=2  OutDataTypeStr=single
  wires:
  Object_Age/1 -> Compare To Constant2/1
  CutInProb/1 -> Switch1/3
  Switch1/1 -> CutInProb_ScopeConstraint/1  "CutInProb_ScopeConstraint"
  [PIL_ObjectCutinMindFlg_ObserVale] -> PIL_ObjectCutinMindFlg_ObserVale/1
  Abs/1 -> Compare To Constant1/1
  PP_ObjectToCenterLine_dy/1 -> Abs/1
  PP_ObjectToCenterLine_vyc/1 -> CutInObjCutoutMov/1(PP_ObjectToCenterLine_vyc)
  ObjectToCenterLine_dy/1 -> CutInObjWidthConstraint/1(ObjectToCenterLine_dy), CutInObjCutoutMov/2(ObjectToCenterLine_dy)
  Object_Width/1 -> CutInObjWidthConstraint/2(Object_Width)
  Compare To Constant1/1 -> Logical Operator2/1
  Compare To Constant2/1 -> Logical Operator2/2
  CutInObjCutoutMov/1(CutInObjCutoutMovflg) -> Logical Operator2/3
  CutInObjWidthConstraint/1(CutInPredictDis_dy_ObjWidthConstraint) -> Logical Operator2/4
  Logical Operator2/1 -> [PIL_ObjectCutinMindFlg_ObserVale], Switch1/2
  C_CutInProb_Val_Zero/1 -> Switch1/1
  Abs1/1 -> Compare To Constant3/1
  PP_ObjectToCenterLine_vyc1/1 -> Abs1/1
  Compare To Constant3/1 -> Terminator/1

== system PubIfDecisionTOS_MDL/TOS_20201112/TOS_2012080320/PIL_1029/ObjCutInOut_Prob/ObjectCutIn/CutInProb_Calculate/CutInProb_Calculate_/CutInProb_ScopeConstraint1 ==
  note: cut in 可能性计算范围约束
  note: cut in 计算概率值约束
  CutInProb : Inport  OutDataTypeStr=single
  PP_ObjectToCenterLine_vyc : Inport  Port=2  OutDataTypeStr=single
  ObjectToCenterLine_dy : Inport  Port=3  OutDataTypeStr=single
  PP_ObjectToCenterLine_dy : Inport  Port=4
  Object_DX : Inport  Port=5  OutDataTypeStr=single
  Object_Age : Inport  Port=6
  Object_Width : Inport  Port=7
  C_CutInProb_Val_Zero : Constant  Value=C_TOS_CutInProb_Val_Zero  OutDataTypeStr=single
      settings: AttributesFormatString=C_TOS_CutInProb_Val_Zero = 0
  C_CutInProb_Val_Zero1 : Constant  Value=C_TOS_CutInProb_Val_Zero  OutDataTypeStr=single
      settings: AttributesFormatString=C_TOS_CutInProb_Val_Zero = 0
  ObjectCutinMind1 : Subsystem
  ScopeConstraint : Subsystem
  Switch : Switch  Criteria=u2 > Threshold  OutDataTypeStr=single
  Switch2 : Switch  Criteria=u2 > Threshold  OutDataTypeStr=single
  PIL_ObjectCutinMindFlg_ObserVale : Outport  OutDataTypeStr=boolean
  CutInProb_ScopeConstraint : Outport  Port=2  OutDataTypeStr=single
  wires:
  [PIL_ObjectCutinMindFlg_ObserVale] -> PIL_ObjectCutinMindFlg_ObserVale/1
  Object_Width/1 -> ObjectCutinMind1/3(Object_Width)
  ObjectToCenterLine_dy/1 -> ObjectCutinMind1/2(ObjectToCenterLine_dy)
  ObjectCutinMind1/1(ObjectCutinMindFlg) -> Switch/2, [PIL_ObjectCutinMindFlg_ObserVale]
  Switch/1 -> CutInProb_ScopeConstraint/1  "CutInProb_ScopeConstraint"
  CutInProb/1 -> Switch2/3
  Switch2/1 -> Switch/3
  C_CutInProb_Val_Zero1/1 -> Switch2/1
  C_CutInProb_Val_Zero/1 -> Switch/1
  PP_ObjectToCenterLine_vyc/1 -> ObjectCutinMind1/1(PP_ObjectToCenterLine_vyc)
  Object_DX/1 -> ScopeConstraint/1(Object_DX)
  PP_ObjectToCenterLine_dy/1 -> ScopeConstraint/2(PP_ObjectToCenterLine_dy)
  Object_Age/1 -> ScopeConstraint/3(Object_Age)
  ScopeConstraint/1(ScopeConstraint) -> Switch2/2
